simulink model "speedgoat_test_IO131"  (R2019a)
settings: Solver=FixedStepDiscrete  StartTime=0.0  StopTime=stop_time  FixedStep=ts  RelTol=1e-3  EnableMultiTasking=on
PreLoadFcn:
  | %ts = 0.001;
  | %sin_base_freq = 1;
  | %ampl = 6;
  | %if ~exist('Ts', 'var')
  | %end
  | %if ~exist('FPGA_Frequency', 'var')
  | %FPGA_Frequency = 33000000;
  | %end
InitFcn:
  | %ts = 0.001;
  | %sin_base_freq = 1;
  | %ampl = 6;
  | %if ~exist('Ts', 'var')
  | %end
  | %if ~exist('FPGA_Frequency', 'var')
  | %FPGA_Frequency = 33000000;
  | %end
values from neighbouring files (symbols this model uses):
  ampl = 1    [main_sim_131.m]
  fs = 10e3    (= 10000)    [main_sim_131.m]
  sin_base_freq = 1    [main_sim_131.m]
  stop_time = 5    [main_sim_131.m]
  ts = 1/fs    (= 0.0001)    [main_sim_131.m]
libraries: speedgoatlib_IO131 x3, slrtlib x1, simulink x1
settings Model: sg_rtwmakecfg_data=_sglibc_  SimulationMode=external  Creator=lab  LastModifiedBy=Admin
settings SolverCC: ConcurrentTasks=on  AutoInsertRateTranBlk=on
settings DataIOCC: SaveFormat=StructureWithTime  ReturnWorkspaceOutputs=off
settings OptimizationCC: BlockReduction=off  OptimizeBlockIOStorage=off  BufferReuse=off  GlobalBufferReuse=off  ExpressionFolding=off  LocalBlockOutputs=off  OptimizeDataStoreBuffers=off  BusAssignmentInplaceUpdate=off
settings DebuggingCC: UnconnectedInputMsg=none  UnconnectedOutputMsg=none  UnconnectedLineMsg=none  PregeneratedLibrarySubsystemCodeDiagnostic=none  ArithmeticOperatorsInVariantConditions=warning
settings HardwareCC: ProdBitPerPointer=32  ProdBitPerSizeT=32  ProdBitPerPtrDiffT=32  ProdLargestAtomicFloat=None  ProdWordSize=32  ProdLongLongMode=on  ProdHWDeviceType=Generic->32-bit x86 compatible
settings SFSimCC: SimUseLocalCustomCode=off
settings RTWCC: SystemTargetFile=slrt.tlc  TemplateMakefile=slrt_default_tmf  Description=Simulink Real-Time  RTWUseLocalCustomCode=off  CodeExecutionProfiling=on  RTWCompilerOptimization=on
settings SimulinkRealTimeCC: SupportVariableSizeSignals=on  PreserveStateflowLocalDataDimensions=off  RL32LogBufSizeModifier=1e8  xPCConcurrentTasks=on

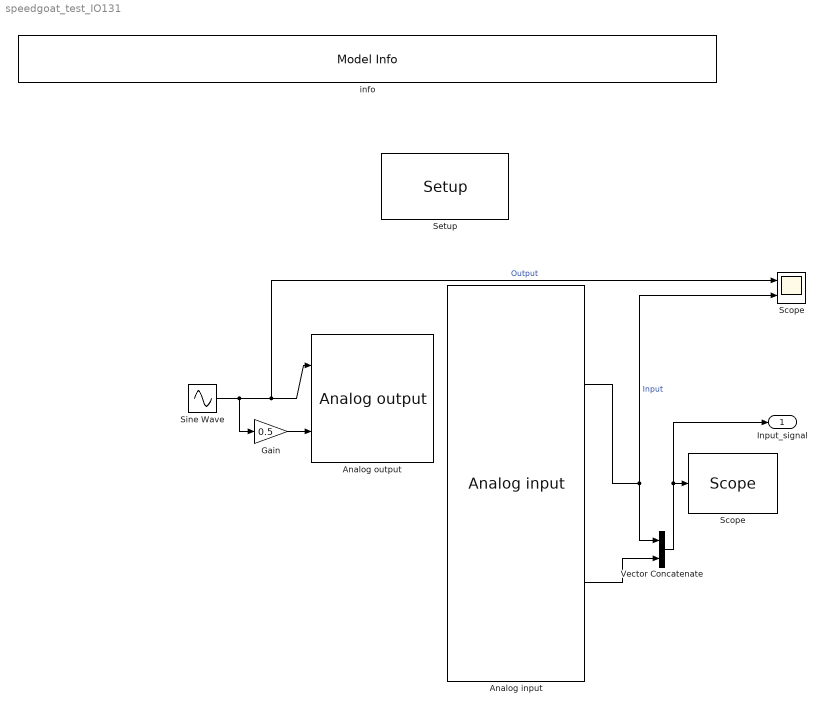
== system speedgoat_test_IO131 ==
  "Analog input " : speedgoatlib_IO131/Analog input   parModuleId=1  parSampleTime=ts  parPciSlot=-1  parRange=+-5V  parOversampling=None  parChannels=[7 16]  parContinuousSampling=off  parDmaEn=off  parDmaChannels=All  parDmaConversionTime=100  parDmaFrameSize=128  parBoardType=131  parIsInitialized=on
      settings: SourceProductName=Simulink Real-Time: Speedgoat I/O Driver Library
  "Analog output " : speedgoatlib_IO131/Analog output   parModuleId=1  parSampleTime=ts  parPciSlot=-1  parRange=+-5V  parChannels=[1 8]  parInitValues=[0 0]  parResetValues=[1 1]  parDmaChannels=All  parDmaEn=off  parDmaClkSrc=2  parDmaConversionTime=100  parDmaFrameSize=128  parBoardType=131  parDoInterrupt=on  parLatency=As small as possible  parIsInitialized=on
      settings: SourceProductName=Simulink Real-Time: Speedgoat I/O Driver Library
  Gain : Gain  Gain=0.5
  Scope : Scope  NumInputPorts=2
  "Scope " : slrtlib/Displays and Logging/Scope   scopeno=1  scopetype=Target  autostart=on  viewmode=Graphical rolling  formatstr='%15.6f'  grid=on  ylimits=[0,0]  nosamples=round(fs*stop_time)  noprepostsamples=0  interleave=1  triggermode=FreeRun  triggersignal=1  trigsignalfromport=off  triggerlevel=0.0  triggerslope=Either  triggerscope=1  triggersample=0  filename=data.dat  mode=Lazy  writesize=512  autorestart=off  dynamicfilemode=off  maxwritefilesize=512*1024^2
  "Setup " : speedgoatlib_IO131/Setup   parPciSlot=-1  parModuleId=1  parTriggerInitiator=Independent  parAdChannels=[7 16]  parAdRange=+-5V  parAdOversampling=None  parAdContinuousSampling=off  parAdDmaEn=off  parAdDmaChannels=All  parAdSampleClock=100e3  parAdDmaFrameSize=128  parAdSampleTime=0.00128  parDaChannels=[1 8]  parDaRange=+-5V  parDaInitValues=[0]  parDaResetValues=[1]  parDaDmaEn=off  parDaDmaChannels=All  parLatency=As small as possible  parDaSampleClock=100000  parClockLocked=off  parDaDmaFrameSize=128  parDaSampleTime=0.00128  parBoardType=131  parForceRefresh=11[]
      settings: SourceProductName=Simulink Real-Time: Speedgoat I/O Driver Library
  Sine Wave : Sin  Amplitude=ampl  Frequency=2*pi*sin_base_freq  SampleTime=ts
  Vector Concatenate : Concatenate
  info : simulink/Model-Wide Utilities/Model Info  Frame=on  DisplayStringWithTags="SPEEDGOAT Simulink Real-Time  test model for Real-time target machine (4684)"  HorizontalTextAlignment=Left  LeftAlignmentValue=0.02
  Input_signal : Outport
  wires:
  Sine Wave/1 -> Scope/1, "Analog output "/1, Gain/1  "Output"
  "Analog input "/1 -> Scope/2, Vector Concatenate/1  "Input"
  "Analog input "/2 -> Vector Concatenate/2
  Vector Concatenate/1 -> Input_signal/1, "Scope "/1
  Gain/1 -> "Analog output "/2
